simulink model "modelqr"  (R2023b)
settings: Solver=VariableStepAuto  StartTime=0.0  StopTime=15  MaxStep=0.1  RelTol=1e-3
values from neighbouring files (symbols this model uses):
  A = double(A_linear)    [main.m]    (also in rlqr.m = [0 1; -6 -5])
  B = double(B_linear)    [main.m]    (also in rlqr.m = [0;1])
  C = eye(2)    [main.m]    (also in rlqr.m)
  D = [0; 0]    [main.m]    (also in rlqr.m = [0;0])
  K = lqr(A, B, Q, R)    [main.m]    (also in rlqr.m = [K11 K12; K12 K23])
  m_val = 1    [main.m]
  u_val = 0.5    [main.m]
settings Model: Creator=ralex  LastModifiedBy=ralex

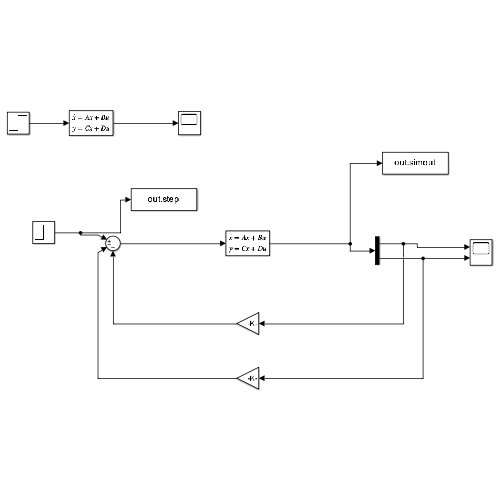
[thumbnail: Simulink's stored preview of the top-level diagram]
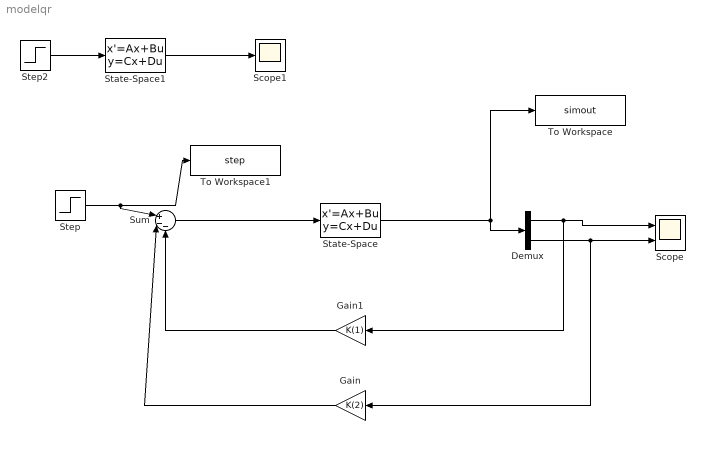
== system modelqr ==
  Demux : Demux  Outputs=2
  Gain : Gain  Gain=K(2)
  Gain1 : Gain  Gain=K(1)
  Scope : Scope  NumInputPorts=2
  Scope1 : Scope
  State-Space : StateSpace  A=A  B=B  C=C  D=D  InitialCondition=[0.5 0.5]
  State-Space1 : StateSpace  A=A  B=B  C=C  D=D  InitialCondition=[0.5 0.5]
  Step : Step  Time=3  After=1/m_val*u_val  SampleTime=0
  Step2 : Step  Time=3  After=1/m_val*u_val  SampleTime=0
  Sum : Sum  Inputs=|+--
  To Workspace : ToWorkspace  VariableName=simout  SaveFormat=Timeseries  SampleTime=-1
  To Workspace1 : ToWorkspace  VariableName=step  SaveFormat=Timeseries  SampleTime=-1
  wires:
  Demux/1 -> Gain1/1, Scope/1
  Gain1/1 -> Sum/3
  Gain/1 -> Sum/2
  Sum/1 -> State-Space/1
  State-Space/1 -> To Workspace/1, Demux/1
  Demux/2 -> Gain/1, Scope/2
  State-Space1/1 -> Scope1/1
  Step2/1 -> State-Space1/1
  Step/1 -> To Workspace1/1, Sum/1
